simulink model "step"  (R2015b)
settings: Solver=VariableStepAuto  StartTime=0.0  StopTime=15  RelTol=1e-3
settings Model: Creator=HP  LastModifiedBy=HP

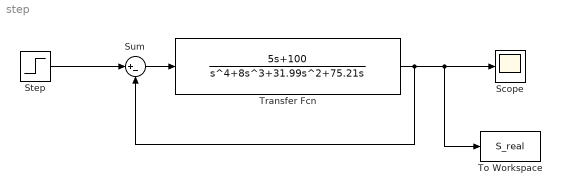
== system step ==
  Scope : Scope
  Step : Step  Time=0  SampleTime=0
  Sum : Sum  Inputs=|+-
  To Workspace : ToWorkspace  VariableName=S_real  SampleTime=0.01
  Transfer Fcn : TransferFcn  Numerator=[0 0 0 5 100]  Denominator=[1 8 31.99 75.21 0]
  wires:
  Sum/1 -> Transfer Fcn/1
  Transfer Fcn/1 -> Sum/2, To Workspace/1, Scope/1
  Step/1 -> Sum/1
